simulink model "chenEx3p3p3mdlV3"  (R2014a)
settings: Solver=ode3  StartTime=0.0  StopTime=TSIM  FixedStep=0.05  RelTol=1e-3
values from neighbouring files (symbols this model uses):
  A = [-3.6         0       0   0 ... (first row only)    [chenEx3p3p3V3.m]
  B = [ 1 0 0 ... (first row only)    [chenEx3p3p3V3.m]
  C = [1    0   0   0 ... (first row only)    [chenEx3p3p3V3.m]
  C1 = C    [chenEx3p3p3V3.m]
  C2 = C    [chenEx3p3p3V3.m]
  C3 = C    [chenEx3p3p3V3.m]
  E = [1;20.758;0;0]    [chenEx3p3p3V3.m]
  F = A1-k1*C    [chenEx3p3p3V3.m]
  F1 = T1*A-k1*C    [chenEx3p3p3V3.m]
  F2 = T2*A-k2*C    [chenEx3p3p3V3.m]
  F3 = T3*A-k2*C    [chenEx3p3p3V3.m]
  fa_u1 = 1    [chenEx3p3p3V3.m]
  fa_u2 = 0    [chenEx3p3p3V3.m]
  fa_u3 = 0    [chenEx3p3p3V3.m]
  faTime = 4    [chenEx3p3p3V3.m]
  faVal = .2*u1Val    (= 6.9264)    [chenEx3p3p3V3.m]
  fsTime = 7    [chenEx3p3p3V3.m]
  fsVal = 0    [chenEx3p3p3V3.m]
  H = E*inv((C*E)'*(C*E))*(C*E)'    [chenEx3p3p3V3.m]
  H1 = E1*inv((C*E1)'*(C*E1))*(C*E1)'    [chenEx3p3p3V3.m]
  H2 = E2*inv((C*E2)'*(C*E2))*(C*E2)'    [chenEx3p3p3V3.m]
  H3 = E3*inv((C*E3)'*(C*E3))*(C*E3)'    [chenEx3p3p3V3.m]
  k = k1 + F*H    [chenEx3p3p3V3.m]
  K1 = k1+F1*H1    [chenEx3p3p3V3.m]
  K2 = k2+F2*H2    [chenEx3p3p3V3.m]
  K3 = k3+F3*H3    [chenEx3p3p3V3.m]
  T = eye(4)-H*C    [chenEx3p3p3V3.m]
  T1 = eye(4) - H1*C    [chenEx3p3p3V3.m]
  T2 = eye(4) - H2*C    [chenEx3p3p3V3.m]
  T3 = eye(4) - H3*C    [chenEx3p3p3V3.m]
  u1Val = 34.632    [chenEx3p3p3V3.m]
  u2Val = 1641.6    [chenEx3p3p3V3.m]
  u3Val = 29980    [chenEx3p3p3V3.m]
  x1_0 = 0.3412    [chenEx3p3p3V3.m]
  x2_0 = 525.7    [chenEx3p3p3V3.m]
  x3_0 = 472.2    [chenEx3p3p3V3.m]
  x4_0 = 496.2    [chenEx3p3p3V3.m]
settings Model: Creator=Sam Nazari  LastModifiedBy=samnazari
settings DataIOCC: SignalLoggingSaveFormat=ModelDataLogs
settings OptimizationCC: InitFltsAndDblsToZero=on
settings DebuggingCC: SaveWithParameterizedLinksMsg=none  UnderspecifiedInitializationDetection=Classic  SignalResolutionControl=TryResolveAllWithWarning  MultiTaskDSMMsg=warning  MultiTaskCondExecSysMsg=none
settings RTWCC: IncludeERTFirstTime=on
settings GRTTargetCC: TargetFcnLib=ansi_tfl_tmw.mat  CombineOutputUpdateFcns=off  GRTInterface=on

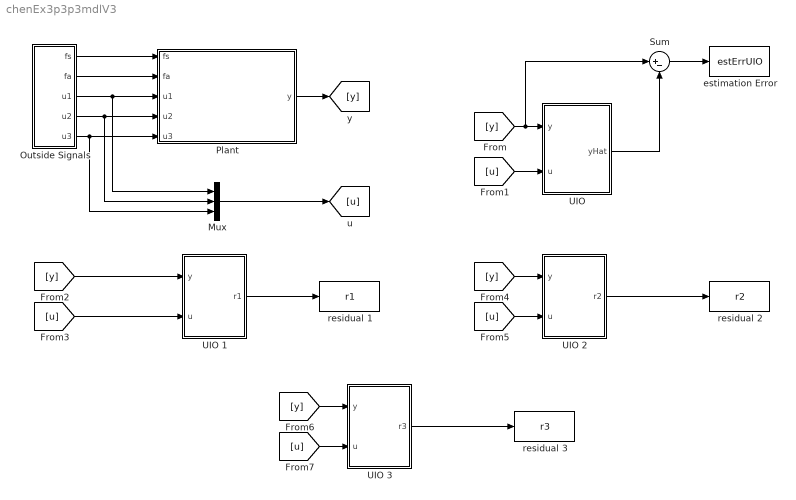
== system chenEx3p3p3mdlV3 ==
  Mux : Mux  Inputs=3
  Outside Signals : Subsystem
  "Plant " : Subsystem
  Sum : Sum  Inputs=|+-
  UIO : Subsystem
  UIO 1 : Subsystem
  UIO 2 : Subsystem
  UIO 3 : Subsystem
  estimation Error : ToWorkspace  VariableName=estErrUIO  SampleTime=-1
  residual 1 : ToWorkspace  VariableName=r1  SampleTime=-1
  residual 2 : ToWorkspace  VariableName=r2  SampleTime=-1
  residual 3 : ToWorkspace  VariableName=r3  SampleTime=-1
  wires:
  UIO/1("yHat ") -> Sum/2
  Sum/1 -> estimation Error/1
  Outside Signals/3("u1 ") -> Mux/1, "Plant "/3(u1)
  Outside Signals/4(u2) -> Mux/2, "Plant "/4(u2)
  Outside Signals/5(u3) -> Mux/3, "Plant "/5(u3)
  Outside Signals/2(fa) -> "Plant "/2(fa)
  "Plant "/1(y) -> [y]
  Mux/1 -> [u]
  [y] -> Sum/1, UIO/1(y)
  [u] -> UIO/2(u)
  [y] -> UIO 1/1(y)
  [u] -> UIO 1/2(u)
  UIO 1/1(r1) -> residual 1/1
  Outside Signals/1(fs) -> "Plant "/1(fs)
  [y] -> UIO 2/1(y)
  [u] -> UIO 2/2(u)
  UIO 2/1(r2) -> residual 2/1
  [y] -> UIO 3/1(y)
  [u] -> UIO 3/2(u)
  UIO 3/1(r3) -> residual 3/1

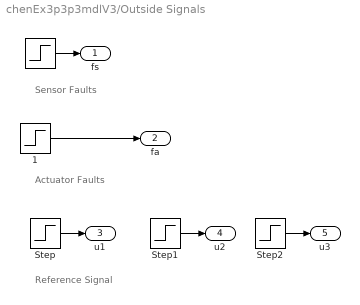
== system chenEx3p3p3mdlV3/Outside Signals ==
  note: Actuator Faults
  note: Sensor Faults
  note: Reference Signal
  "  " : Step  Time=fsTime  After=fsVal  SampleTime=0
  "  1" : Step  Time=faTime  After=faVal  SampleTime=0
  Step : Step  Time=0  After=u1Val  SampleTime=0
  Step1 : Step  Time=0  After=u2Val  SampleTime=0
  Step2 : Step  Time=0  After=u3Val  SampleTime=0
  fs : Outport
  fa : Outport  Port=2
  "u1 " : Outport  Port=3
  u2 : Outport  Port=4
  u3 : Outport  Port=5
  wires:
  "  "/1 -> fs/1
  Step/1 -> "u1 "/1
  Step1/1 -> u2/1
  Step2/1 -> u3/1
  "  1"/1 -> fa/1

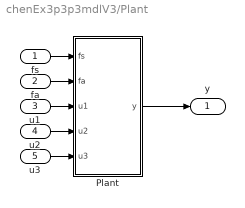
== system chenEx3p3p3mdlV3/Plant  ==
  fs : Inport
  fa : Inport  Port=2
  u1 : Inport  Port=3
  u2 : Inport  Port=4
  u3 : Inport  Port=5
  Plant : Subsystem
  y : Outport
  wires:
  Plant/1(y) -> y/1
  fa/1 -> Plant/2(fa)
  fs/1 -> Plant/1(fs)
  u1/1 -> Plant/3(u1)
  u2/1 -> Plant/4(u2)
  u3/1 -> Plant/5(u3)

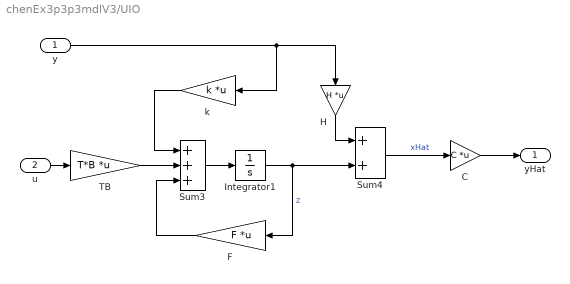
== system chenEx3p3p3mdlV3/UIO ==
  y : Inport
  u : Inport  Port=2
  C : Gain  Gain=C  Multiplication=Matrix(K*u)
  F : Gain  Gain=F  Multiplication=Matrix(K*u)
  H : Gain  Gain=H  Multiplication=Matrix(K*u)
  Integrator1 : Integrator
  Sum3 : Sum  Inputs=+++
  Sum4 : Sum
  TB : Gain  Gain=T*B  Multiplication=Matrix(K*u)
  k : Gain  Gain=k  Multiplication=Matrix(K*u)
  "yHat " : Outport
  wires:
  Sum3/1 -> Integrator1/1
  Integrator1/1 -> F/1, Sum4/2  "z"
  F/1 -> Sum3/3
  k/1 -> Sum3/1
  TB/1 -> Sum3/2
  H/1 -> Sum4/1
  Sum4/1 -> C/1  "xHat"
  y/1 -> H/1, k/1
  u/1 -> TB/1
  C/1 -> "yHat "/1

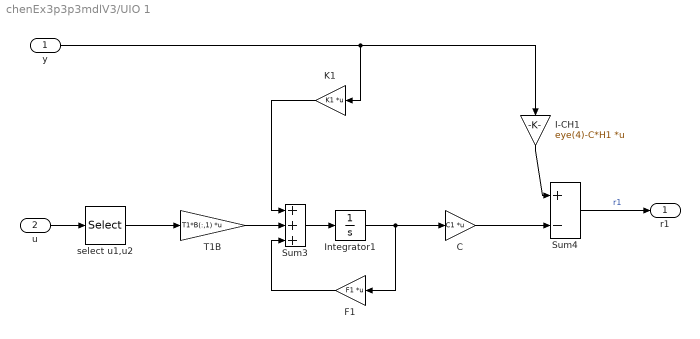
== system chenEx3p3p3mdlV3/UIO 1 ==
  y : Inport
  u : Inport  Port=2
  C : Gain  Gain=C1  Multiplication=Matrix(K*u)
  F1 : Gain  Gain=F1  Multiplication=Matrix(K*u)
  I-CH1 : Gain  Gain=eye(4)-C*H1  Multiplication=Matrix(K*u)
  Integrator1 : Integrator
  K1 : Gain  Gain=K1  Multiplication=Matrix(K*u)
  Sum3 : Sum  Inputs=+++
  Sum4 : Sum  Inputs=+-
  T1B : Gain  Gain=T1*B(:,1)  Multiplication=Matrix(K*u)
  select u1,u2 : Selector  InputPortWidth=3
  r1 : Outport
  wires:
  Sum3/1 -> Integrator1/1
  Integrator1/1 -> C/1, F1/1
  F1/1 -> Sum3/3
  K1/1 -> Sum3/1
  T1B/1 -> Sum3/2
  Sum4/1 -> r1/1  "r1"
  y/1 -> I-CH1/1, K1/1
  I-CH1/1 -> Sum4/1
  C/1 -> Sum4/2
  select u1,u2/1 -> T1B/1
  u/1 -> select u1,u2/1

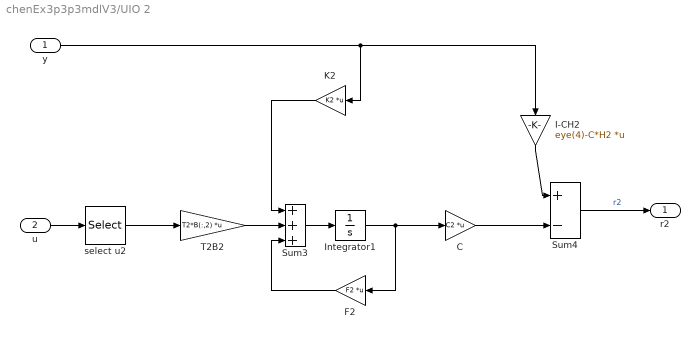
== system chenEx3p3p3mdlV3/UIO 2 ==
  y : Inport
  u : Inport  Port=2
  C : Gain  Gain=C2  Multiplication=Matrix(K*u)
  F2 : Gain  Gain=F2  Multiplication=Matrix(K*u)
  I-CH2 : Gain  Gain=eye(4)-C*H2  Multiplication=Matrix(K*u)
  Integrator1 : Integrator
  K2 : Gain  Gain=K2  Multiplication=Matrix(K*u)
  Sum3 : Sum  Inputs=+++
  Sum4 : Sum  Inputs=+-
  T2B2 : Gain  Gain=T2*B(:,2)  Multiplication=Matrix(K*u)
  select u2 : Selector  InputPortWidth=3  Indices=2
  r2 : Outport
  wires:
  u/1 -> select u2/1
  select u2/1 -> T2B2/1
  C/1 -> Sum4/2
  I-CH2/1 -> Sum4/1
  y/1 -> K2/1, I-CH2/1
  Sum4/1 -> r2/1  "r2"
  T2B2/1 -> Sum3/2
  K2/1 -> Sum3/1
  F2/1 -> Sum3/3
  Integrator1/1 -> F2/1, C/1
  Sum3/1 -> Integrator1/1

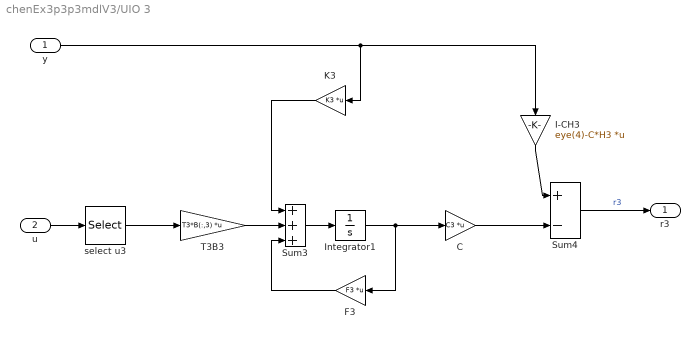
== system chenEx3p3p3mdlV3/UIO 3 ==
  y : Inport
  u : Inport  Port=2
  C : Gain  Gain=C3  Multiplication=Matrix(K*u)
  F3 : Gain  Gain=F3  Multiplication=Matrix(K*u)
  I-CH3 : Gain  Gain=eye(4)-C*H3  Multiplication=Matrix(K*u)
  Integrator1 : Integrator
  K3 : Gain  Gain=K3  Multiplication=Matrix(K*u)
  Sum3 : Sum  Inputs=+++
  Sum4 : Sum  Inputs=+-
  T3B3 : Gain  Gain=T3*B(:,3)  Multiplication=Matrix(K*u)
  select u3 : Selector  InputPortWidth=3  Indices=3
  r3 : Outport
  wires:
  u/1 -> select u3/1
  select u3/1 -> T3B3/1
  C/1 -> Sum4/2
  I-CH3/1 -> Sum4/1
  y/1 -> K3/1, I-CH3/1
  Sum4/1 -> r3/1  "r3"
  T3B3/1 -> Sum3/2
  K3/1 -> Sum3/1
  F3/1 -> Sum3/3
  Integrator1/1 -> F3/1, C/1
  Sum3/1 -> Integrator1/1

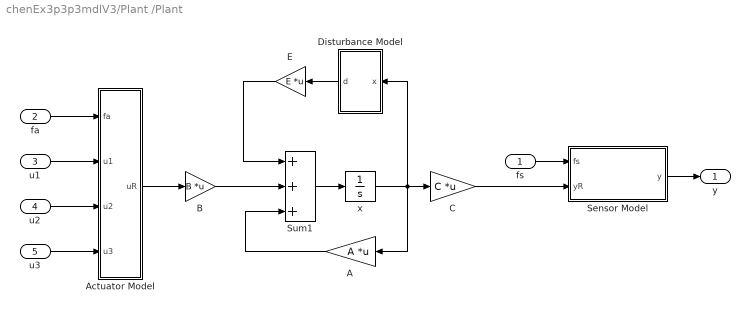
== system chenEx3p3p3mdlV3/Plant /Plant ==
  fs : Inport
  fa : Inport  Port=2
  u1 : Inport  Port=3
  u2 : Inport  Port=4
  u3 : Inport  Port=5
  A : Gain  Gain=A  Multiplication=Matrix(K*u)
  Actuator Model : Subsystem
  B : Gain  Gain=B  Multiplication=Matrix(K*u) (u vector)
  C : Gain  Gain=C  Multiplication=Matrix(K*u)
  Disturbance Model : Subsystem
  E : Gain  Gain=E  Multiplication=Matrix(K*u)
  Sensor Model : Subsystem
  Sum1 : Sum  Inputs=+++
  x : Integrator  InitialCondition=[x1_0;x2_0;x3_0;x4_0]
  y : Outport
  wires:
  Sum1/1 -> x/1
  x/1 -> Disturbance Model/1(x), C/1, A/1
  A/1 -> Sum1/3
  E/1 -> Sum1/1
  fs/1 -> Sensor Model/1(fs)
  C/1 -> Sensor Model/2(yR)
  Sensor Model/1(y) -> y/1
  fa/1 -> Actuator Model/1(fa)
  Actuator Model/1(uR) -> B/1
  Disturbance Model/1(d) -> E/1
  u1/1 -> Actuator Model/2(u1)
  u2/1 -> Actuator Model/3(u2)
  u3/1 -> Actuator Model/4(u3)
  B/1 -> Sum1/2

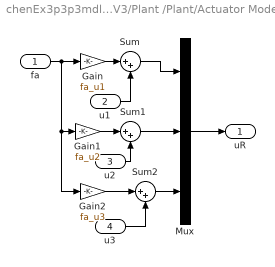
== system chenEx3p3p3mdlV3/Plant /Plant/Actuator Model ==
  fa : Inport
  u1 : Inport  Port=2
  u2 : Inport  Port=3
  u3 : Inport  Port=4
  Gain : Gain  Gain=fa_u1
  Gain1 : Gain  Gain=fa_u2
  Gain2 : Gain  Gain=fa_u3
  Mux : Mux  Inputs=3
  Sum : Sum  Inputs=|++
  Sum1 : Sum  Inputs=|++
  Sum2 : Sum  Inputs=|++
  uR : Outport
  wires:
  u1/1 -> Sum/2
  fa/1 -> Gain2/1, Gain1/1, Gain/1
  Mux/1 -> uR/1
  Sum/1 -> Mux/1
  Gain/1 -> Sum/1
  Gain1/1 -> Sum1/1
  u2/1 -> Sum1/2
  Sum1/1 -> Mux/2
  Gain2/1 -> Sum2/1
  u3/1 -> Sum2/2
  Sum2/1 -> Mux/3

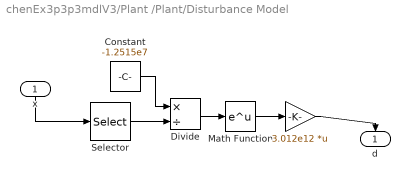
== system chenEx3p3p3mdlV3/Plant /Plant/Disturbance Model ==
  x : Inport
  "  " : Gain  Gain=3.012e12  Multiplication=Matrix(K*u)
  Constant : Constant  Value=-1.2515e7
  Divide : Product  Inputs=*/
  Math Function : Math  SaturateOnIntegerOverflow=on
  Selector : Selector  InputPortWidth=4  Indices=2
  d : Outport
  wires:
  Selector/1 -> Divide/2
  Constant/1 -> Divide/1
  Divide/1 -> Math Function/1
  Math Function/1 -> "  "/1
  "  "/1 -> d/1
  x/1 -> Selector/1

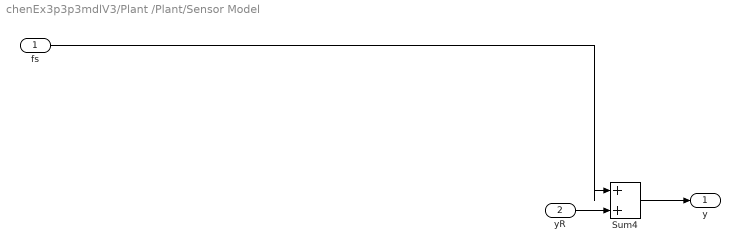
== system chenEx3p3p3mdlV3/Plant /Plant/Sensor Model ==
  fs : Inport
  yR : Inport  Port=2
  Sum4 : Sum  Inputs=|++
  y : Outport
  wires:
  yR/1 -> Sum4/2
  Sum4/1 -> y/1
  fs/1 -> Sum4/1
